simulink model "MotorXploer"  (R2024b)
settings: Solver=VariableStepAuto  StartTime=0.0  StopTime=inf  RelTol=1e-3
undefined symbols (not defined in the file): Blocking, LF, Non
libraries: hdlsllib x5, amg_usbconverter_n_connect_lib x3
settings Model: Creator=beamk  LastModifiedBy=beamk

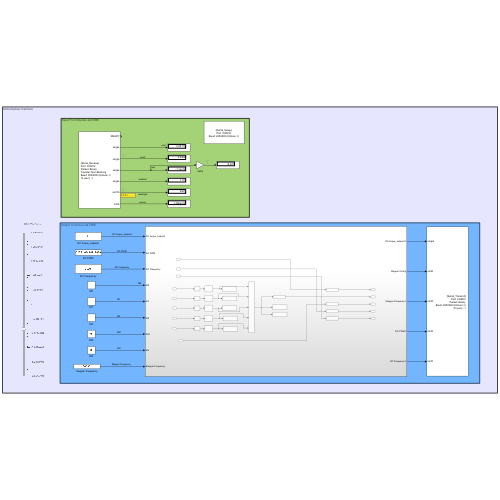
[thumbnail: Simulink's stored preview of the top-level diagram]
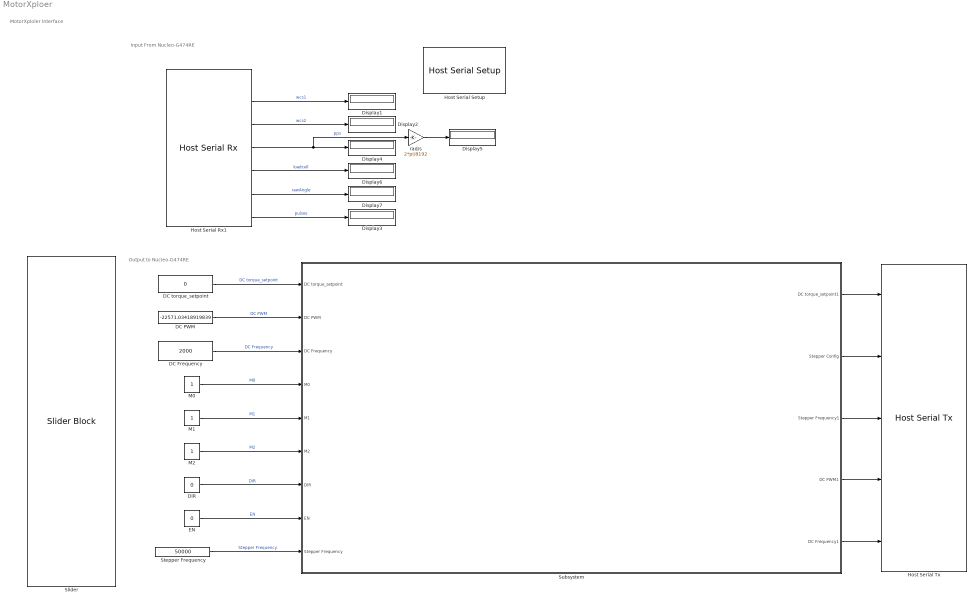
== system MotorXploer ==
  note: Output to Nucleo-G474RE
  note: Input From Nucleo-G474RE
  note: MotorXploler Interface
  DC Frequency : Constant  Value=2000
  DC PWM : Constant  Value=-22571.03418919839
  DC torque_setpoint : Constant  Value=0
  DIR : Constant  Value=0  OutDataTypeStr=uint8
  Display{1..7} (7 alike) : Display
  EN : Constant  Value=0  OutDataTypeStr=uint8
  Host Serial Rx1 : amg_usbconverter_n_connect_lib/Host Serial Rx  conf=rx  port=<auto>  baudrate=2000000  databits=8  parity=None  stopbit=1  flowcontrol=None  transfer=Non-Blocking  timeout=5  packetmode=Binary  enableinitialvalues=off  initialvalues=[]  binheader='45'  binterminator='A'  porttype_double=0  porttype_single=4  porttype_int8=0  porttype_uint8=0  porttype_int16=0  porttype_uint16=1  porttype_int32=1  porttype_uint32=0  asciiformat='%f,%f,%d,%d'  rx_asciiterminator="LF (0x0A - \"\\n\")"  tx_asciiterminator="CRLF (0x0D 0x0A - \"\\r\\n\")"  sampletime=-1  enablecustomportlabel=off  cinputportlabel=0  coutputportlabel=A  portpinstr=0  blockid=HostSerialRx1  inputporttype=[]  inputportwidth=[]  inputportlabel={}  outputporttype=[3 1 1 1 1 5 6]  outputportwidth=[1 1 1 1 1 1 1]  outputportlabel={'READY','single','single','single','single','uint16','int32'}  compat=0  optionstring=[]  autoport='COM12'
  Host Serial Setup : amg_usbconverter_n_connect_lib/Host Serial Setup  conf=setup  port=<auto>  baudrate=2000000  databits=8  parity=None  stopbit=1  flowcontrol=None  transfer=Blocking  timeout=2  packetmode=Binary  initialvalues=[]  binheader='7E 7E'  binterminator='03 03'  porttype_double=0  porttype_single=1  porttype_int8=0  porttype_uint8=0  porttype_int16=0  porttype_uint16=0  porttype_int32=0  porttype_uint32=2  asciiformat='%d %u %x'  rx_asciiterminator="CRLF (0x0D 0x0A - \"\\r\\n\")"  tx_asciiterminator="CRLF (0x0D 0x0A - \"\\r\\n\")"  sampletime=-1  enablecustomportlabel=off  cinputportlabel=0  coutputportlabel=A  portpinstr=0  blockid=HostSerialSetup  inputporttype=[]  inputportwidth=[]  inputportlabel={}  outputporttype=[]  outputportwidth=[]  outputportlabel={}  compat=0  optionstring=[]  autoport='COM12'
  Host Serial Tx : amg_usbconverter_n_connect_lib/Host Serial Tx  conf=tx  port=<auto>  baudrate=2000000  databits=8  parity=None  stopbit=1  flowcontrol=None  transfer=Blocking  timeout=2  packetmode=Binary  initialvalues=[]  binheader='45'  binterminator='A'  porttype_double=0  porttype_single=1  porttype_int8=0  porttype_uint8=1  porttype_int16=0  porttype_uint16=0  porttype_int32=3  porttype_uint32=0  asciiformat='%d,%f'  rx_asciiterminator="CRLF (0x0D 0x0A - \"\\r\\n\")"  tx_asciiterminator="CRLF (0x0D 0x0A - \"\\r\\n\")"  sampletime=-1  enablecustomportlabel=off  cinputportlabel=0  coutputportlabel=A  portpinstr=0  blockid=HostSerialTx  inputporttype=[1 3 6 6 6]  inputportwidth=[1 1 1 1 1]  inputportlabel={'single','uint8','int32','int32','int32'}  outputporttype=[]  outputportwidth=[]  outputportlabel={}  compat=0  optionstring=[]  autoport='COM12'
      settings: SourceProductName=aMG USB Converter N
  M0 : Constant  OutDataTypeStr=uint8
  M1 : Constant  OutDataTypeStr=uint8
  M2 : Constant  OutDataTypeStr=uint8
  Slider : SliderBlock  ScaleMin=-65535  ScaleMax=65535
  Stepper Frequency : Constant  Value=50000
  Subsystem : Subsystem
  rad/s : Gain  Gain=2*pi/8192
  wires:
  rad/s/1 -> Display5/1
  Host Serial Rx1/7 -> Display3/1  "pulses"
  Host Serial Rx1/2 -> Display1/1  "wcs1"
  Host Serial Rx1/4 -> Display4/1, rad/s/1  "pps"
  Host Serial Rx1/3 -> Display2/1  "wcs2"
  Host Serial Rx1/5 -> Display6/1  "loadcell"
  Host Serial Rx1/6 -> Display7/1  "rawAngle"
  DC torque_setpoint/1 -> Subsystem/1(DC torque_setpoint)  "DC torque_setpoint"
  DC PWM/1 -> Subsystem/2(DC PWM)  "DC PWM"
  DC Frequency/1 -> Subsystem/3(DC Frequency)  "DC Frequency"
  M0/1 -> Subsystem/4(M0)  "M0"
  M1/1 -> Subsystem/5(M1)  "M1"
  M2/1 -> Subsystem/6(M2)  "M2"
  DIR/1 -> Subsystem/7(DIR)  "DIR"
  EN/1 -> Subsystem/8(EN)  "EN"
  Stepper Frequency/1 -> Subsystem/9(Stepper Frequency)  "Stepper Frequency"
  Subsystem/1(DC torque_setpoint1) -> Host Serial Tx/1
  Subsystem/2(Stepper Config) -> Host Serial Tx/2
  Subsystem/3(Stepper Frequency1) -> Host Serial Tx/3
  Subsystem/4(DC PWM1) -> Host Serial Tx/4
  Subsystem/5(DC Frequency1) -> Host Serial Tx/5

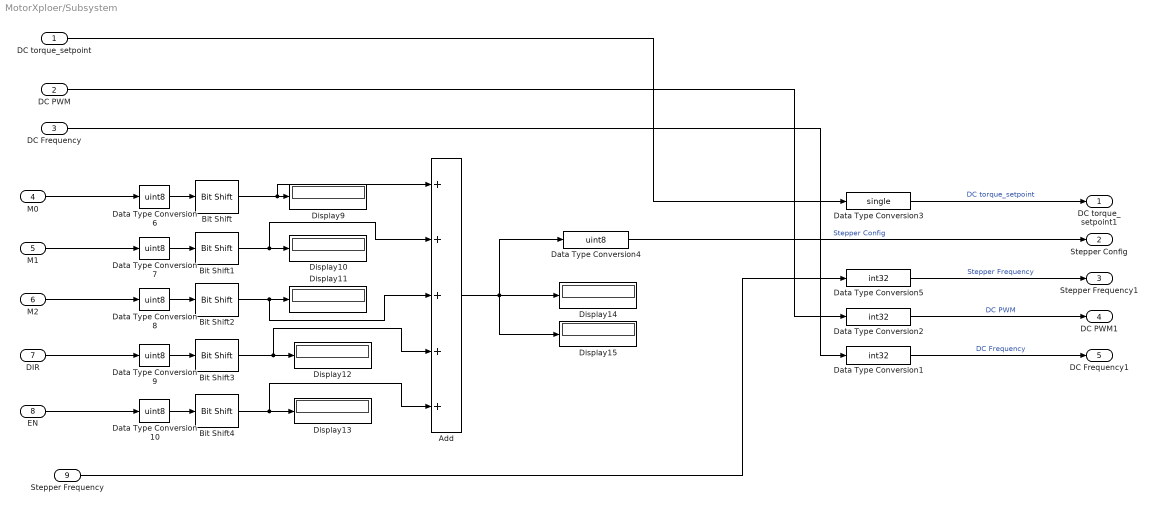
== system MotorXploer/Subsystem ==
  DC torque_setpoint : Inport
  DC PWM : Inport  Port=2
  DC Frequency : Inport  Port=3
  M0 : Inport  Port=4
  M1 : Inport  Port=5
  M2 : Inport  Port=6
  DIR : Inport  Port=7
  EN : Inport  Port=8
  Stepper Frequency : Inport  Port=9
  Add : Sum  Inputs=+++++
  Bit Shift : hdlsllib/Logic and Bit Operations/Bit Shift  mode=Shift Left Logical  N=4
  Bit Shift1 : hdlsllib/Logic and Bit Operations/Bit Shift  mode=Shift Left Logical  N=3
  Bit Shift2 : hdlsllib/Logic and Bit Operations/Bit Shift  mode=Shift Left Logical  N=2
  Bit Shift3 : hdlsllib/Logic and Bit Operations/Bit Shift  mode=Shift Left Logical  N=1
  Bit Shift4 : hdlsllib/Logic and Bit Operations/Bit Shift  mode=Shift Left Logical  N=0
  Data Type Conversion1 : DataTypeConversion  OutDataTypeStr=int32  SaturateOnIntegerOverflow=off  RndMeth=Floor
  Data Type Conversion{4,6..10} (6 alike) : DataTypeConversion  OutDataTypeStr=uint8  SaturateOnIntegerOverflow=off  RndMeth=Floor
  Data Type Conversion2 : DataTypeConversion  OutDataTypeStr=int32  SaturateOnIntegerOverflow=off  RndMeth=Floor
  Data Type Conversion3 : DataTypeConversion  OutDataTypeStr=single  SaturateOnIntegerOverflow=off  RndMeth=Floor
  Data Type Conversion5 : DataTypeConversion  OutDataTypeStr=int32  SaturateOnIntegerOverflow=off  RndMeth=Floor
  Display{9..15} (7 alike) : Display
      Display10 settings: Format=binary (Stored Integer)
      Display11 settings: Format=binary (Stored Integer)
      Display12 settings: Format=binary (Stored Integer)
      Display13 settings: Format=binary (Stored Integer)
      Display14 settings: Format=binary (Stored Integer)
      Display9 settings: Format=binary (Stored Integer)
  DC torque_setpoint1 : Outport
  Stepper Config : Outport  Port=2
  Stepper Frequency1 : Outport  Port=3
  DC PWM1 : Outport  Port=4
  DC Frequency1 : Outport  Port=5
  wires:
  Add/1 -> Data Type Conversion4/1, Display14/1, Display15/1
  M2/1 -> Data Type Conversion8/1
  DC Frequency/1 -> Data Type Conversion1/1
  Bit Shift3/1 -> Add/4, Display12/1
  Stepper Frequency/1 -> Data Type Conversion5/1
  Bit Shift2/1 -> Add/3, Display11/1
  Data Type Conversion7/1 -> Bit Shift1/1
  Data Type Conversion4/1 -> Stepper Config/1  "Stepper Config"
  Bit Shift/1 -> Add/1, Display9/1
  Data Type Conversion6/1 -> Bit Shift/1
  Data Type Conversion1/1 -> DC Frequency1/1  "DC Frequency"
  Data Type Conversion10/1 -> Bit Shift4/1
  Data Type Conversion2/1 -> DC PWM1/1  "DC PWM"
  Bit Shift4/1 -> Add/5, Display13/1
  Data Type Conversion8/1 -> Bit Shift2/1
  Data Type Conversion3/1 -> DC torque_setpoint1/1  "DC torque_setpoint"
  EN/1 -> Data Type Conversion10/1
  M0/1 -> Data Type Conversion6/1
  Bit Shift1/1 -> Add/2, Display10/1
  Data Type Conversion9/1 -> Bit Shift3/1
  DIR/1 -> Data Type Conversion9/1
  DC torque_setpoint/1 -> Data Type Conversion3/1
  DC PWM/1 -> Data Type Conversion2/1
  M1/1 -> Data Type Conversion7/1
  Data Type Conversion5/1 -> Stepper Frequency1/1  "Stepper Frequency"
